simulink model "Tut15_EnableSubsystem"  (R2021a)
settings: Solver=FixedStepDiscrete  StartTime=0.0  StopTime=10.0  FixedStep=1  RelTol=1e-3
settings Model: Creator=cheta  LastModifiedBy=cheta

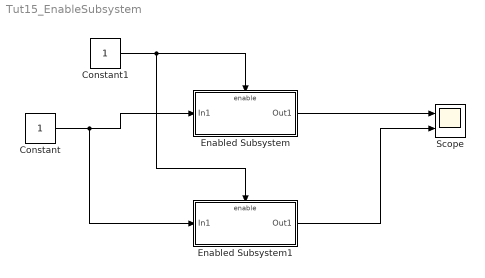
== system Tut15_EnableSubsystem ==
  Constant : Constant
  Constant1 : Constant  OutDataTypeStr=boolean
  Enabled Subsystem : Subsystem  TreatAsAtomicUnit=on
  Enabled Subsystem1 : Subsystem  TreatAsAtomicUnit=on
  Scope : Scope  NumInputPorts=2
  wires:
  Constant/1 -> Enabled Subsystem1/1(In1), Enabled Subsystem/1(In1)
  Constant1/1 -> Enabled Subsystem1/Enable, Enabled Subsystem/Enable
  Enabled Subsystem/1(Out1) -> Scope/1
  Enabled Subsystem1/1(Out1) -> Scope/2

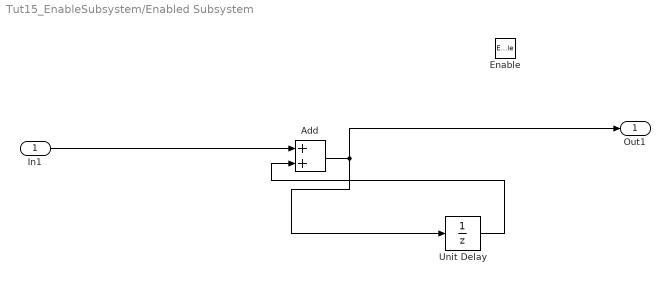
== system Tut15_EnableSubsystem/Enabled Subsystem ==
  In1 : Inport
  Enable : EnablePort
  Add : Sum
  Unit Delay : UnitDelay  SampleTime=-1  HasFrameUpgradeWarning=on
  Out1 : Outport
  wires:
  In1/1 -> Add/1
  Add/1 -> Out1/1, Unit Delay/1
  Unit Delay/1 -> Add/2

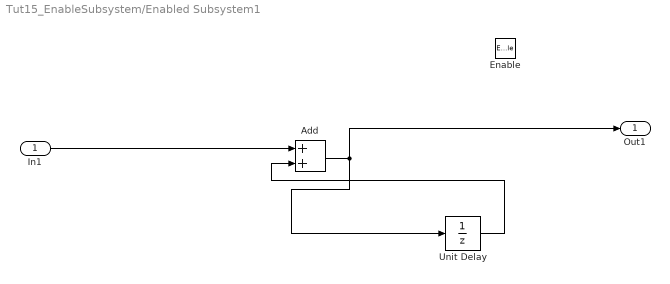
== system Tut15_EnableSubsystem/Enabled Subsystem1 ==
  In1 : Inport
  Enable : EnablePort  StatesWhenEnabling=reset
  Add : Sum
  Unit Delay : UnitDelay  SampleTime=-1  HasFrameUpgradeWarning=on
  Out1 : Outport
  wires:
  Unit Delay/1 -> Add/2
  Add/1 -> Unit Delay/1, Out1/1
  In1/1 -> Add/1
